simulink model "TestPulsoMotores"  (R2023b)
settings: Solver=FixedStepAuto  StartTime=0.0  StopTime=10.0  RelTol=1e-3  EnableMultiTasking=on
libraries: SignalEditorBlockLib x1
settings Model: ExtModeTrigDuration=2  Creator=Enrique  LastModifiedBy=Enrique
settings OptimizationCC: EnhancedBackFolding=on  PassReuseOutputArgsAs=Individual arguments  ZeroExternalMemoryAtStartup=off  ZeroInternalMemoryAtStartup=off  MaxStackSize=64  OptimizeBlockOrder=speed  DifferentSizesBufferReuse=on  OptimizationCustomize=off  EfficientTunableParamExpr=on
settings DebuggingCC: ParameterTunabilityLossMsg=error
settings HardwareCC: ProdBitPerInt=16  ProdBitPerPointer=16  ProdBitPerSizeT=16  ProdBitPerPtrDiffT=16  ProdLargestAtomicFloat=None  ProdWordSize=8  ProdHWDeviceType=Atmel->AVR  UseEmbeddedCoderFeatures=off  UseSimulinkCoderFeatures=off
settings SFSimCC: MATLABDynamicMemAlloc=off
settings RTWCC: Description=Embedded Coder  SystemTargetFile=ert.tlc  HardwareBoard=Arduino Mega 2560  TemplateMakefile=ert_default_tmf  Toolchain=Arduino AVR  BuildConfiguration=Faster Runs
settings CodeAppCC: ForceParamTrailComments=on  IgnoreCustomStorageClasses=off  OperatorAnnotations=on  SimulinkDataObjDesc=on  SFDataObjDesc=on  InsertBlockDesc=on
settings ERTTargetCC: SupportContinuousTime=on  SupportNonInlinedSFcns=on  SupportVariableSizeSignals=on  ExtModeTransport=3  ExtModeStaticAlloc=on  ExtModeAutomaticAllocSize=off  ExtModeStaticAllocSize=2048  ExtModeMexFile=ext_xcp  ExtModeIntrfLevel=Level2 - Open

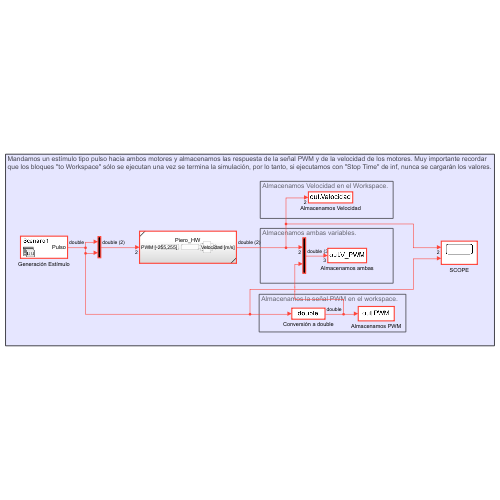
[thumbnail: Simulink's stored preview of the top-level diagram]
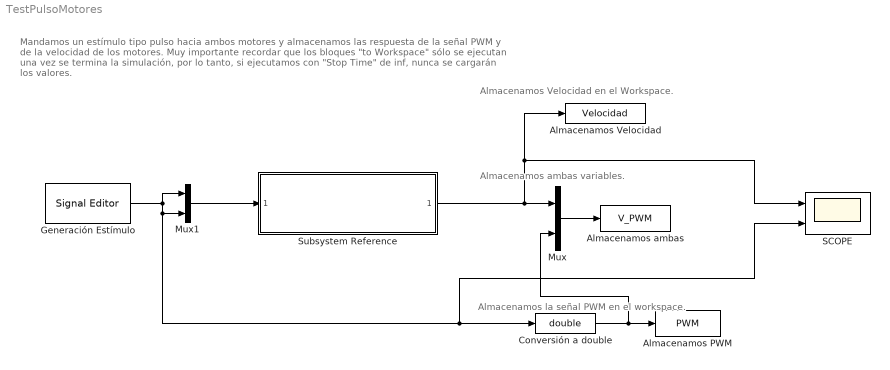
== system TestPulsoMotores ==
  note: Mandamos un estímulo tipo pulso hacia ambos motores y almacenamos las respuesta de la señal PWM y de la velocidad de los motores. Muy importante recordar
      | que los bloques "to Workspace" sólo se ejecutan una vez se termina la simulación, por lo tanto, si ejecutamos con "Stop Time" de inf, nunca se cargarán los valores.
  note: Almacenamos ambas variables.
  note: Almacenamos Velocidad en el Workspace.
  note: Almacenamos la señal PWM en el workspace.
  Almacenamos PWM : ToWorkspace  VariableName=PWM  SampleTime=-1
      settings: Save2DSignal=2-D array (concatenate along first dimension)
  Almacenamos Velocidad : ToWorkspace  VariableName=Velocidad  SampleTime=-1
      settings: Save2DSignal=2-D array (concatenate along first dimension)
  Almacenamos ambas : ToWorkspace  VariableName=V_PWM  SampleTime=-1
      settings: Save2DSignal=2-D array (concatenate along first dimension)
  Conversión a double : DataTypeConversion  OutDataTypeStr=double  SaturateOnIntegerOverflow=off  RndMeth=Floor
  Generación Estímulo : SignalEditorBlockLib/Signal Editor  FileName=C:\Users\Enrique\MATLAB\Projects\EnriqueGF10\Piero\Datos Señales\Rampa.mat  ActiveScenario=Scenario1  ActiveSignal=Pulso  IsBus=off  OutputBusObjectStr=Bus: BusObject  SampleTime=0.01  Interpolate=off  ZeroCross=off  OutputAfterFinalValue=Setting to zero  Unit=inherit  PreserveSignalName=on  ApplySigPropsToAllScenarios=on  ApplySigPropsToAllSignals=off
  Mux : Mux  Inputs=2
  Mux1 : Mux  Inputs=2
  SCOPE : Scope  NumInputPorts=2
  Subsystem Reference : Subsystem  ReferencedSubsystem=Piero_HW
  wires:
  Subsystem Reference/1 -> Almacenamos Velocidad/1, SCOPE/1, Mux/1
  Conversión a double/1 -> Mux/2, Almacenamos PWM/1
  Mux/1 -> Almacenamos ambas/1
  Generación Estímulo/1 -> SCOPE/2, Conversión a double/1, Mux1/2, Mux1/1
  Mux1/1 -> Subsystem Reference/1
